simulink model "sfcndemo_io_handling_ada"  (Simulink 6.0)
settings: Solver=FixedStepDiscrete  StartTime=0.0  StopTime=10.0  RelTol=1e-3
PreLoadFcn:
  | t=0;u=[1 2 3 4 5 0 0 0 0 0 0 0 0 0 0];
undefined symbols (not defined in the file or in its folder): DiscIntNeverNeededParam
settings Model: Creator=The MathWorks Inc.  LastModifiedBy=batserve  ExtModeAutoUpdateStatusClock=off
settings DataIOCC: LoadExternalInput=on  SaveState=on
settings OptimizationCC: BlockReduction=off  BooleanDataType=off  InlineInvariantSignals=off
settings DebuggingCC: CheckExecutionContextPreStartOutputMsg=on  CheckExecutionContextRuntimeOutputMsg=on  SolverPrmCheckMsg=none
settings HardwareCC: TargetUnknown=on
settings RTWCC: SystemTargetFile=rt_ada_sim.tlc  MakeCommand=make_rtw -ada=gnat3.12a2  TemplateMakefile=gnat_sim.tmf  RetainRTWFile=on  ProcessScript=rt_ada_sim_make_rtw_hook
settings STFCustomTargetCC: TargetFcnLib=ansi_tfl_tmw.mat  GenFloatMathFcnCalls=ANSI_C  ModelReferenceCompliant=off  CombineOutputUpdateFcns=on  MatFileLogging=on  SystemTargetFile=rt_ada_sim.tlc

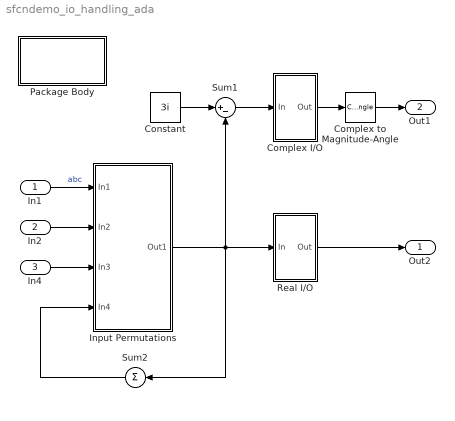
== system sfcndemo_io_handling_ada ==
  In1 : Inport  Port=1  PortDimensions=5  LatchInput=off
  In2 : Inport  Port=2  PortDimensions=5  LatchInput=off
  In4 : Inport  Port=3  PortDimensions=5  LatchInput=off
      settings: SignalType=complex
  Complex I/O : Subsystem  PropExecContextAcrossSSBoundary=on
  Complex to Magnitude-Angle : ComplexToMagnitudeAngle  Output=Magnitude
  Constant : Constant  Value=3i
  Input Permutations : Subsystem  PropExecContextAcrossSSBoundary=on
  Package Body : Subsystem  PropExecContextAcrossSSBoundary=on
      settings: CopyFcn=cccopyfcn(gcb)  OpenFcn=accopenfcn('Package Body')
      mask Type: Package Body
      mask Description: Add code to model .adb file
      mask Help: This block contains text fields to insert custom user code at the package body level.  You can add with dependencies, declarations, and elaboration code to the package body (models.adb file).
      mask Display: disp('Package\nBody');
  Real I/O : Subsystem  PropExecContextAcrossSSBoundary=on
  Sum1 : Sum  Inputs=|+-  SaturateOnIntegerOverflow=on  InputSameDT=on
  Sum2 : Sum  Orientation=left  Inputs=+  SaturateOnIntegerOverflow=on  InputSameDT=on
  Out2 : Outport
  Out1 : Outport  Port=2
  wires:
  In1/1 -> Input Permutations/1(In1)  "abc"
  In4/1 -> Input Permutations/3(In3)
  Sum2/1 -> Input Permutations/4(In4)
  Complex I/O/1(Out) -> Complex to Magnitude-Angle/1
  In2/1 -> Input Permutations/2(In2)
  Input Permutations/1(Out1) -> Real I/O/1(In), Sum2/1, Sum1/2
  Real I/O/1(Out) -> Out2/1
  Complex to Magnitude-Angle/1 -> Out1/1
  Sum1/1 -> Complex I/O/1(In)
  Constant/1 -> Sum1/1

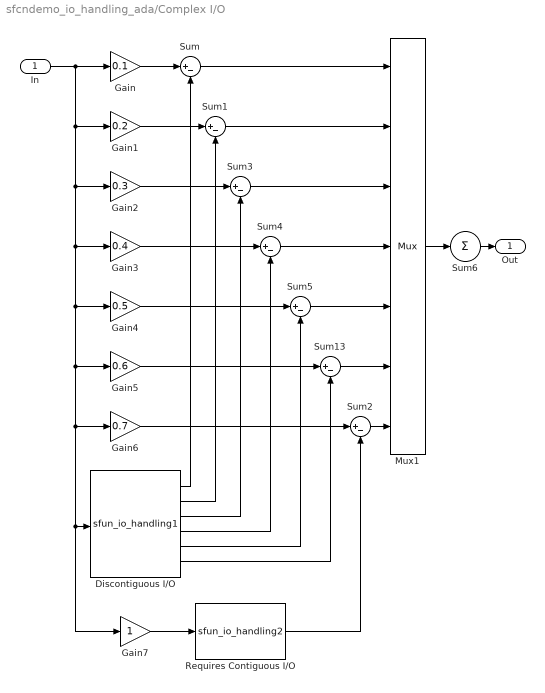
== system sfcndemo_io_handling_ada/Complex I/O ==
  In : Inport  Port=1  LatchInput=off
  Discontiguous I/O : S-Function  FunctionName=sfun_io_handling1
  Gain : Gain  Gain=0.1  SaturateOnIntegerOverflow=on
  Gain1 : Gain  Gain=0.2  SaturateOnIntegerOverflow=on
  Gain2 : Gain  Gain=0.3  SaturateOnIntegerOverflow=on
  Gain3 : Gain  Gain=0.4  SaturateOnIntegerOverflow=on
  Gain4 : Gain  Gain=0.5  SaturateOnIntegerOverflow=on
  Gain5 : Gain  Gain=0.6  SaturateOnIntegerOverflow=on
  Gain6 : Gain  Gain=0.7  SaturateOnIntegerOverflow=on
  Gain7 : Gain  SaturateOnIntegerOverflow=on
  Mux1 : Mux  Inputs=7
  Requires Contiguous I/O : S-Function  FunctionName=sfun_io_handling2
  Sum{,1..5,13} (7 alike) : Sum  Inputs=|+-  SaturateOnIntegerOverflow=on  InputSameDT=on
  Sum6 : Sum  Inputs=+  SaturateOnIntegerOverflow=on  InputSameDT=on
  Out : Outport
  wires:
  Gain7/1 -> Requires Contiguous I/O/1
  Gain/1 -> Sum/1
  Gain1/1 -> Sum1/1
  Discontiguous I/O/1 -> Sum/2
  Discontiguous I/O/2 -> Sum1/2
  Gain2/1 -> Sum3/1
  Discontiguous I/O/3 -> Sum3/2
  Gain3/1 -> Sum4/1
  Gain4/1 -> Sum5/1
  Discontiguous I/O/4 -> Sum4/2
  Discontiguous I/O/5 -> Sum5/2
  Sum6/1 -> Out/1
  Sum/1 -> Mux1/1
  Sum1/1 -> Mux1/2
  Sum3/1 -> Mux1/3
  Sum4/1 -> Mux1/4
  Sum5/1 -> Mux1/5
  Mux1/1 -> Sum6/1
  Sum13/1 -> Mux1/6
  Gain5/1 -> Sum13/1
  Discontiguous I/O/6 -> Sum13/2
  In/1 -> Gain/1, Gain1/1, Gain2/1, Gain3/1, Gain4/1, Gain5/1, Gain7/1, Discontiguous I/O/1, Gain6/1
  Gain6/1 -> Sum2/1
  Sum2/1 -> Mux1/7
  Requires Contiguous I/O/1 -> Sum2/2

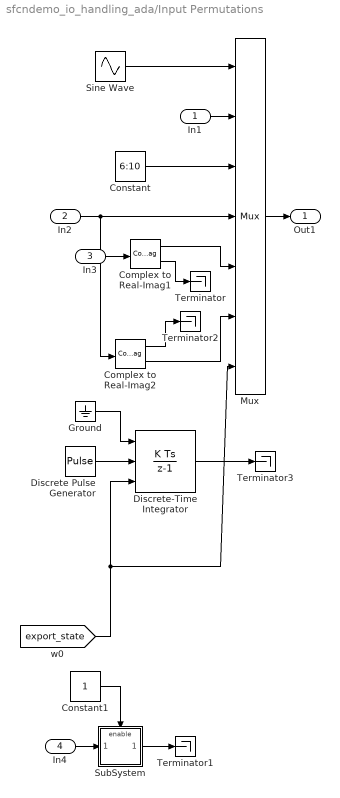
== system sfcndemo_io_handling_ada/Input Permutations ==
  In1 : Inport  Port=1  LatchInput=off
  In2 : Inport  Port=2  LatchInput=off
  In3 : Inport  Port=3  LatchInput=off
  In4 : Inport  Port=4  LatchInput=off
  Complex to Real-Imag1 : ComplexToRealImag
  Complex to Real-Imag2 : ComplexToRealImag
  Constant : Constant  Value=6:10
  Constant1 : Constant
  Discrete Pulse Generator : DiscretePulseGenerator
  Discrete-Time Integrator : DiscreteIntegrator  ExternalReset=either  InitialConditionSource=external  InitialCondition=-5:-1  ICPrevOutput=DiscIntNeverNeededParam  ICPrevScaledInput=DiscIntNeverNeededParam
  Ground : Ground
  Mux : Mux  Inputs=7
  Sine Wave : Sin  Amplitude=1:5  SampleTime=1
  SubSystem : Subsystem  TreatAsAtomicUnit=on  PropExecContextAcrossSSBoundary=on
  Terminator{,1..3} (4 alike) : Terminator
  Out1 : Outport
  wires:
  Sine Wave/1 -> Mux/1
  Constant/1 -> Mux/3
  Constant1/1 -> SubSystem/Enable
  [export_state] -> Discrete-Time Integrator/3, Mux/7
  Discrete Pulse Generator/1 -> Discrete-Time Integrator/2
  Complex to Real-Imag1/1 -> Mux/5
  Complex to Real-Imag2/2 -> Mux/6
  SubSystem/1(Out1) -> Terminator1/1
  Complex to Real-Imag1/2 -> Terminator/1
  Complex to Real-Imag2/1 -> Terminator2/1
  Ground/1 -> Discrete-Time Integrator/1
  Discrete-Time Integrator/1 -> Terminator3/1
  In1/1 -> Mux/2
  In2/1 -> Mux/4, Complex to Real-Imag2/1
  Mux/1 -> Out1/1
  In3/1 -> Complex to Real-Imag1/1
  In4/1 -> SubSystem/1(In1)

== system sfcndemo_io_handling_ada/Package Body ==

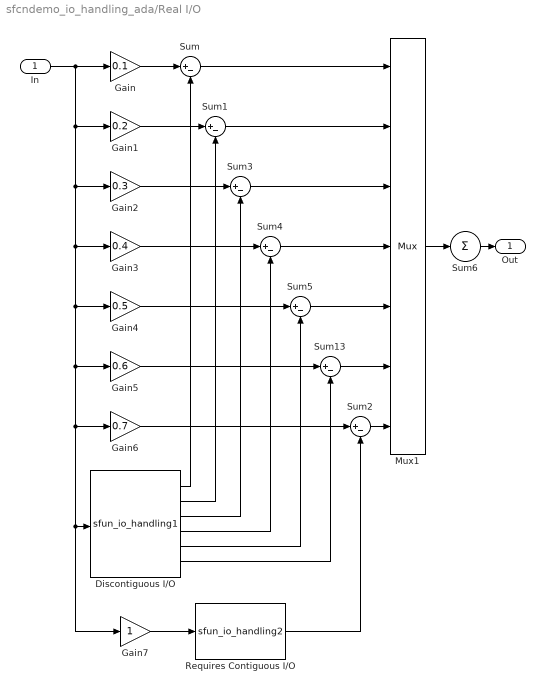
== system sfcndemo_io_handling_ada/Real I/O ==
  In : Inport  Port=1  LatchInput=off
  Discontiguous I/O : S-Function  FunctionName=sfun_io_handling1
  Gain : Gain  Gain=0.1  SaturateOnIntegerOverflow=on
  Gain1 : Gain  Gain=0.2  SaturateOnIntegerOverflow=on
  Gain2 : Gain  Gain=0.3  SaturateOnIntegerOverflow=on
  Gain3 : Gain  Gain=0.4  SaturateOnIntegerOverflow=on
  Gain4 : Gain  Gain=0.5  SaturateOnIntegerOverflow=on
  Gain5 : Gain  Gain=0.6  SaturateOnIntegerOverflow=on
  Gain6 : Gain  Gain=0.7  SaturateOnIntegerOverflow=on
  Gain7 : Gain  SaturateOnIntegerOverflow=on
  Mux1 : Mux  Inputs=7
  Requires Contiguous I/O : S-Function  FunctionName=sfun_io_handling2
  Sum{,1..5,13} (7 alike) : Sum  Inputs=|+-  SaturateOnIntegerOverflow=on  InputSameDT=on
  Sum6 : Sum  Inputs=+  SaturateOnIntegerOverflow=on  InputSameDT=on
  Out : Outport
  wires:
  Requires Contiguous I/O/1 -> Sum2/2
  Sum2/1 -> Mux1/7
  Gain6/1 -> Sum2/1
  In/1 -> Gain6/1, Discontiguous I/O/1, Gain7/1, Gain5/1, Gain4/1, Gain3/1, Gain2/1, Gain1/1, Gain/1
  Discontiguous I/O/6 -> Sum13/2
  Gain5/1 -> Sum13/1
  Sum13/1 -> Mux1/6
  Mux1/1 -> Sum6/1
  Sum5/1 -> Mux1/5
  Sum4/1 -> Mux1/4
  Sum3/1 -> Mux1/3
  Sum1/1 -> Mux1/2
  Sum/1 -> Mux1/1
  Sum6/1 -> Out/1
  Discontiguous I/O/5 -> Sum5/2
  Discontiguous I/O/4 -> Sum4/2
  Gain4/1 -> Sum5/1
  Gain3/1 -> Sum4/1
  Discontiguous I/O/3 -> Sum3/2
  Gain2/1 -> Sum3/1
  Discontiguous I/O/2 -> Sum1/2
  Discontiguous I/O/1 -> Sum/2
  Gain1/1 -> Sum1/1
  Gain/1 -> Sum/1
  Gain7/1 -> Requires Contiguous I/O/1

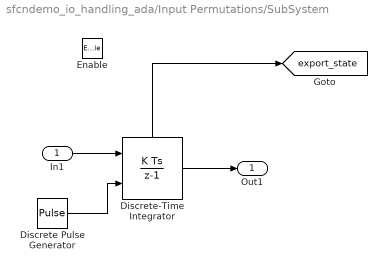
== system sfcndemo_io_handling_ada/Input Permutations/SubSystem ==
  In1 : Inport  Port=1  LatchInput=off
  Enable : EnablePort
  Discrete Pulse Generator : DiscretePulseGenerator
  Discrete-Time Integrator : DiscreteIntegrator  ExternalReset=either  InitialCondition=-5:-1  ShowStatePort=on  ICPrevOutput=DiscIntNeverNeededParam  ICPrevScaledInput=DiscIntNeverNeededParam
  Out1 : Outport
  tag scope: export_state=global
  wires:
  In1/1 -> Discrete-Time Integrator/1
  Discrete-Time Integrator/State -> [export_state]
  Discrete Pulse Generator/1 -> Discrete-Time Integrator/2
  Discrete-Time Integrator/1 -> Out1/1
